simulink model "physical_test_voo"  (R2020a)
settings: Solver=FixedStepAuto  StartTime=0.0  StopTime=10.0  FixedStep=1e-3  RelTol=1e-3  EnableMultiTasking=on
undefined symbols (not defined in the file or in its folder): D1, D10, D12, D2, D3, D5, D9, PTA1, PTA2, PTB9, PTC17, PTC4, PTD0, PTD3
libraries: frdmk64flib x9
settings Model: ExtModeTrigDuration=5  Creator=emily  LastModifiedBy=emily
settings OptimizationCC: EnhancedBackFolding=on  PassReuseOutputArgsAs=Individual arguments  ZeroExternalMemoryAtStartup=off  ZeroInternalMemoryAtStartup=off  MaxStackSize=64  OptimizeBlockOrder=speed  DifferentSizesBufferReuse=on  OptimizationCustomize=off  EfficientTunableParamExpr=on
settings DebuggingCC: ParameterTunabilityLossMsg=error
settings HardwareCC: ProdBitPerPointer=32  ProdBitPerSizeT=32  ProdBitPerPtrDiffT=32  ProdLargestAtomicInteger=Long  ProdLargestAtomicFloat=Double  ProdWordSize=32  ProdHWDeviceType=ARM Compatible->ARM Cortex
settings SFSimCC: MATLABDynamicMemAlloc=off
settings RTWCC: SystemTargetFile=ert.tlc  HardwareBoard=NXP FRDM-K64F  TemplateMakefile=ert_default_tmf  Toolchain=GNU Tools for ARM Embedded Processors
settings CodeAppCC: ForceParamTrailComments=on  IgnoreCustomStorageClasses=off  OperatorAnnotations=on  SimulinkDataObjDesc=on  SFDataObjDesc=on  InsertBlockDesc=on

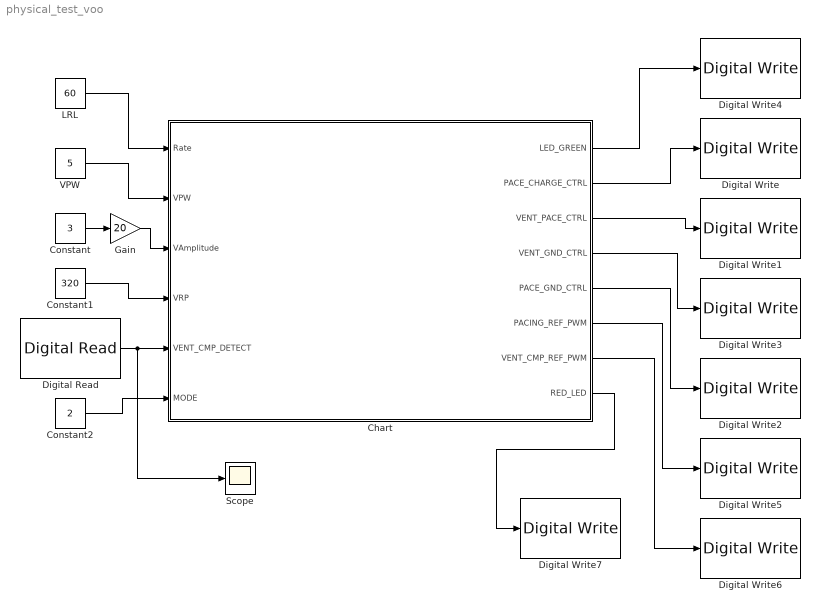
== system physical_test_voo ==
  Chart : Stateflow chart  TreatAsAtomicUnit=on
  Constant : Constant  Value=3
  Constant1 : Constant  Value=320
  Constant2 : Constant  Value=2  OutDataTypeStr=int16
  Digital Read : frdmk64flib/Digital Read  Whichpin=PTC17 (D1)  SampleTime=-1
  Digital Write : frdmk64flib/Digital Write  Whichpin=PTB9 (D2)
  Digital Write1 : frdmk64flib/Digital Write  Whichpin=PTC4 (D9)
  Digital Write2 : frdmk64flib/Digital Write  Whichpin=PTD0 (D10)
  Digital Write3 : frdmk64flib/Digital Write  Whichpin=PTD3 (D12)
  Digital Write4 : frdmk64flib/Digital Write  Whichpin=GREEN_LED
  Digital Write5 : frdmk64flib/Digital Write  Whichpin=PTA2 (D5)
  Digital Write6 : frdmk64flib/Digital Write  Whichpin=PTA1 (D3)
  Digital Write7 : frdmk64flib/Digital Write  Whichpin=RED_LED
  Gain : Gain  Gain=20
  LRL : Constant  Value=60
  Scope : Scope
  VPW : Constant  Value=5
  wires:
  VPW/1 -> Chart/2(VPW)
  LRL/1 -> Chart/1(Rate)
  Chart/5(PACE_GND_CTRL) -> Digital Write2/1
  Chart/4(VENT_GND_CTRL) -> Digital Write3/1
  Chart/3(VENT_PACE_CTRL) -> Digital Write1/1
  Chart/2(PACE_CHARGE_CTRL) -> Digital Write/1
  Chart/1(LED_GREEN) -> Digital Write4/1
  Chart/6(PACING_REF_PWM) -> Digital Write5/1
  Constant/1 -> Gain/1
  Gain/1 -> Chart/3(VAmplitude)
  Constant1/1 -> Chart/4(VRP)
  Constant2/1 -> Chart/6(MODE)
  Digital Read/1 -> Scope/1, Chart/5(VENT_CMP_DETECT)
  Chart/7(VENT_CMP_REF_PWM) -> Digital Write6/1
  Chart/8(RED_LED) -> Digital Write7/1

== stateflow chart physical_test_voo/Chart ==
  state VOO
    entry:
    PACE_GND_CTRL = 1;
    PACING_REF_PWM = VAmplitude;
    state TIMING
      entry:
      LED_GREEN = 0;
      PACE_CHARGE_CTRL =1;
      VENT_PACE_CTRL = 0;
      VENT_GND_CTRL = 1;
    state PULSE
      entry:
      LED_GREEN = 1;
      PACE_CHARGE_CTRL =0;
      VENT_PACE_CTRL = 1;
      VENT_GND_CTRL = 0;
    (default) -> TIMING
    PULSE -> TIMING : after(VPW, msec)
    TIMING -> PULSE : after(60000/Rate -VPW, msec)
  state VVI
    entry:
    PACE_GND_CTRL = 1;
    PACING_REF_PWM = VAmplitude;
    VENT_CMP_REF_PWM=60;
    state WAIT
      entry:
      PACE_CHARGE_CTRL = 1;
      VENT_PACE_CTRL = 0;
      VENT_GND_CTRL = 1;
      RED_LED = 0;
      LED_GREEN = 0;
    state PACE
      entry:
      PACE_CHARGE_CTRL = 0;
      VENT_PACE_CTRL = 1;
      VENT_GND_CTRL = 0;
      RED_LED = 0;
      LED_GREEN = 1;
    state REFRACTORY
      entry:
      PACE_CHARGE_CTRL = 1;
      VENT_PACE_CTRL = 0;
      VENT_GND_CTRL = 1;
      RED_LED = 1;
      LED_GREEN = 0;
    (default) -> WAIT
    WAIT -> PACE [order 1] : after(60000/Rate ,msec)
    WAIT -> REFRACTORY [order 2] : [VENT_CMP_DETECT]
    REFRACTORY -> WAIT : after(VRP, msec)
    PACE -> REFRACTORY : after(VPW,msec)
  (default) -> VVI
  VOO -> VVI : [MODE==2]
  VVI -> VOO : [MODE==1]
  data: Rate input; VPW input; LED_GREEN output int16; PACE_CHARGE_CTRL output int16; VENT_PACE_CTRL output int16; VENT_GND_CTRL output int16; PACE_GND_CTRL output int16; PACING_REF_PWM output double; VAmplitude input double; VRP input; VENT_CMP_DETECT input; MODE input int16; VENT_CMP_REF_PWM output; RED_LED output
